simulink model "Espaco_estados_28_02_24"  (R2023b)
settings: Solver=VariableStepAuto  StartTime=0.0  StopTime=30  RelTol=1e-3
settings Model: Creator=stem  LastModifiedBy=stem

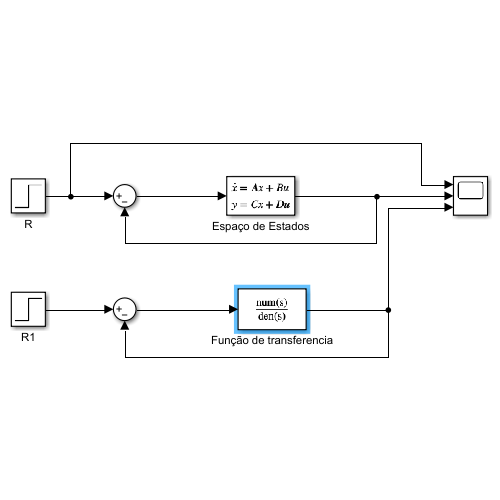
[thumbnail: Simulink's stored preview of the top-level diagram]
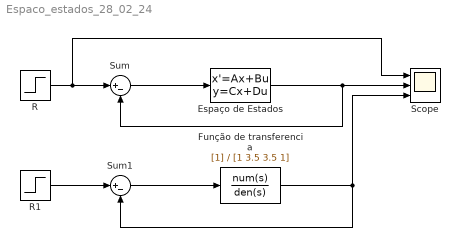
== system Espaco_estados_28_02_24 ==
  Espaço de Estados : StateSpace  A=[-3.5 -3.5 -1 ; 1 0 0; 0 1 0]  B=[1; 0; 0]  C=[0 0 1]  D=0  InitialCondition=0
  Função de transferencia : TransferFcn  Denominator=[1 3.5 3.5 1]
  R : Step  SampleTime=0
  R1 : Step  Time=0.5  SampleTime=0
  Scope : Scope  NumInputPorts=3
  Sum : Sum  Inputs=|+-
  Sum1 : Sum  Inputs=|+-
  wires:
  R/1 -> Scope/1, Sum/1
  Sum/1 -> Espaço de Estados/1
  Espaço de Estados/1 -> Sum/2, Scope/2
  Sum1/1 -> Função de transferencia/1
  Função de transferencia/1 -> Scope/3, Sum1/2
  R1/1 -> Sum1/1
